simulink model "sedemo_gg1"  (Simulink 7.5)
settings: Solver=ode45  StartTime=0.0  StopTime=10000  RelTol=1e-3
PostLoadFcn:
  | open_system([gcs '/Arrival Process Variance']);
  | open_system([gcs '/Service Process Variance']);
  | open_system([gcs '/Queue Content']);
  | open_system([gcs '/Arrival Rate: Theoretical  vs. Simulation Results']);
undefined symbols (not defined in the file or in its folder): des_attributefunction_support, DiscIntNeverNeededParam
libraries: simulink x6, simeventsattributes2 x3, simeventssink1 x1, simeventsqueue1 x1, simeventstranslate1 x1, simeventsinfo x1, simeventsserver1 x1, simeventsgenerators1 x1
CloseFcn:
  | close_system([gcs '/Arrival Process Variance']);
  | close_system([gcs '/Service Process Variance']);
  | close_system([gcs '/Queue Content']);
  | close_system([gcs '/Arrival Rate: Theoretical  vs. Simulation Results']);
settings Model: Creator=The MathWorks Inc.  ExtModeAutoUpdateStatusClock=off
settings DataIOCC: SaveOutput=off  SignalLogging=off  SaveTime=off
settings OptimizationCC: InitFltsAndDblsToZero=on  BufferReusableBoundary=off
settings DebuggingCC: SignalResolutionControl=TryResolveAllWithWarning  SolverPrmCheckMsg=none  MultiTaskDSMMsg=warning  MultiTaskCondExecSysMsg=none  SigSpecEnsureSampleTimeMsg=none  IntegerOverflowMsg=none  Int32ToFloatConvMsg=none  ParameterDowncastMsg=none  ParameterOverflowMsg=none  ParameterPrecisionLossMsg=none  BusObjectLabelMismatch=none  StrictBusMsg=None
settings RTWCC: IncludeERTFirstTime=on
settings SimEventsCC: propIdentEventSeed=12345678  propDiagAttribOutput=1  propDiagFcnCallOutput=1  propDiagStatOutput=0

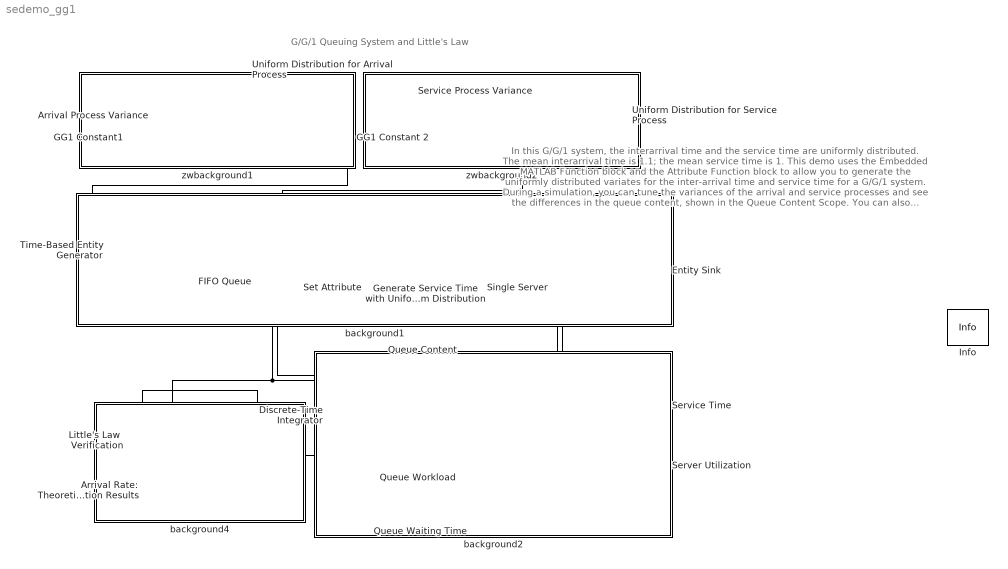
== system sedemo_gg1 ==
  note: G/G/1 Queuing System and Little's Law
  note: In this G/G/1 system, the interarrival time and the
      | service time are uniformly distributed. The mean
      | interarrival time is 1.1; the mean service time is 1.
      |
      | This demo uses the Embedded MATLAB Function
      | block and the Attribute Function block to allow you
      | to generate the  uniformly distributed variates for the
      | inter-arrival time and service time for a G/G/1 system.
      |
      | During a simulation, you can tune the variances of
      | the arrival and service processes and see the
      | differences in the queue content, shown in the Queue
      | Content Scope.
      |
      | You can also verify the Little's law by deriving
      | the arrival rate from average workload and
      | average waiting time. See the Arrival Rate Scope for
      | details.
  Arrival Process Variance : simulink/Math Operations/Slider Gain  SystemSampleTime=-1  low=0  gain=0.3  high=0.40333
  Arrival Rate: Theoretical  vs. Simulation Results : Scope
      settings: YMin=0  YMax=1.1
  Discrete-Time Integrator : DiscreteIntegrator  SampleTime=0.2  OutDataType=sfix(16)  OutScaling=2^0  ICPrevOutput=DiscIntNeverNeededParam  ICPrevScaledInput=DiscIntNeverNeededParam
  Entity Sink : simeventssink1/Entity Sink  Priority=1  SystemSampleTime=-1  AvailableForArrivals=on  StatNumberArrived=Off
  FIFO Queue : simeventsqueue1/FIFO Queue  Priority=1  SystemSampleTime=-1  Capacity=Inf  EnableTOPort=off  StatNumberDeparted=Off  StatNumberInBlock=On  StatPendingEntity=Off  StatAverageWait=On  StatAverageQueueLength=Off  StatNumberTimedout=Off
  "GG1 Constant 2 " : Constant  OutDataType=sfix(16)  OutScaling=2^0
  GG1 Constant1 : Constant  OutDataType=sfix(16)  OutScaling=2^0
  Generate Service Time with Uniform Distribution : Subsystem  LoadFcn=des_attributefunction_support(gcb,'LoadFcn');  StartFcn=des_attributefunction_support(gcb,'StartFcn');  mask(Attribute Function){OutputNamePrefix=out_}
      mask prompts: OutputNamePrefix "Prefix name"
      settings: CopyFcn=des_attributefunction_support(gcb,'CopyFcn');  OpenFcn=des_attributefunction_support(gcb,'OpenFcn');  ErrorFcn=des_error_redirect
      mask Display: image(des_iconLoad('attribFunction.jpg'),'center');
  Info : simeventsinfo/Info  SystemSampleTime=-1
  Little's Law  Verification : Subsystem
      mask Type: Little's Law Evaluation
      mask Description: Evaluate arrival rate from average workload and mean waiting time according to Little's Law. Combine and output this result and the known arrival rate.
      mask Display: disp('Little''s Law\nEvaluation');
  Queue Content : Scope
      settings: YMin=0  YMax=12  SaveName=ScopeData5
  Queue Waiting Time : Display
  Queue Workload : Display
  Server Utilization : Display
  Service Process Variance : simulink/Math Operations/Slider Gain  SystemSampleTime=-1  low=0  gain=0.3  high=0.33333
  Service Time : Display
  Set Attribute : simeventsattributes2/Set Attribute  Priority=1  DialogController=des_ddg_create  DialogControllerArgs=DataTag8  SystemSampleTime=-1  AttributeFrom=Signal port  AttributeName=Variance  AttributeTreatAsVector=1  AttributeValue=1  AttributeCreate=on  StatNumberDeparted=Off  EvaluatedAttributeValue={[]}
  Single Server : simeventsserver1/Single Server  Priority=1  SystemSampleTime=-1  ServiceTimeFrom=Attribute  ServiceTime=1  AttributeName=ServiceTime  PriorityServiceCompletion=1  PermitPreemption=off  SortingAttributeName=PriorityAttributeName  SortingDirection=Ascending  WriteToAttribute=off  ResidualAttributeName=ResidualServiceTime  CreateAttribute=on  EnableTOPort=off  StatNumberDeparted=Off  StatNumberInBlock=Off  StatNumberPreempted=Off  StatPendingEntity=Off  StatAverageWait=On  StatUtilization=On  StatNumberTimedout=Off
  Time-Based Entity Generator : simeventsgenerators1/Entity Generators/Time-Based Entity Generator  Priority=1  DialogController=des_ddg_create  DialogControllerArgs=DataTag11  SystemSampleTime=-1  GenerateEntitiesUpon=Intergeneration time from port t  Distribution=Constant  Minimum=0  Maximum=1  Mean=1  InitialSeed=12345  Period=1  PriorityEntityGeneration=1  GenerateEntityAtSimulationStart=on  ResponseWhenBlocked=Pause generation  ResponseWhenUnblocked=Immediate restart  EntityType=Standard  StatNumberDeparted=Off  StatPendingEntity=Off  StatAverageIntergenerationTime=Off
  Uniform Distribution for Arrival Process : Subsystem  mask(Uniform Distribution for Interarrival Time){seed=85274}
      mask prompts: seed "Initial seed"
      mask help: Output interarrival times according to a uniform distribution. The mean is set to 1.1 and the variance is determined by the input. Output is repeatable for a given seed.
      mask Display: disp('Uniform\nDistribution for\nInterarrival Time');
  Uniform Distribution for Service Process : Subsystem
      mask Display: disp(['Variance ' char(10) 'Validation']);
  background1 : Subsystem
      mask Display: disp('')
  background2 : Subsystem
      mask Display: disp('')
  background4 : Subsystem
      mask Display: disp('')
  zwbackground1 : Subsystem
      mask Display: disp('')
  zwbackground2 : Subsystem
      mask Display: disp('')
  wires:
  FIFO Queue/1 -> Queue Content/1, Discrete-Time Integrator/1
  FIFO Queue/2 -> Queue Waiting Time/1, Little's Law  Verification/2(Waiting Time)
  Arrival Process Variance/1 -> Uniform Distribution for Arrival Process/1(Variance)
  GG1 Constant1/1 -> Arrival Process Variance/1
  Uniform Distribution for Arrival Process/1(Out1) -> Time-Based Entity Generator/1
  Service Process Variance/1 -> Set Attribute/1, Uniform Distribution for Service Process/1(Variance)
  "GG1 Constant 2 "/1 -> Service Process Variance/1
  Discrete-Time Integrator/1 -> Little's Law  Verification/1(Number of  Customers Served), Queue Workload/1
  Single Server/1 -> Service Time/1
  Little's Law  Verification/1(Out1) -> Arrival Rate: Theoretical  vs. Simulation Results/1
  Single Server/2 -> Server Utilization/1
  connections:
  Time-Based Entity Generator/RConn1 -- FIFO Queue/LConn1
  Single Server/RConn1 -- Entity Sink/LConn1
  Set Attribute/LConn1 -- FIFO Queue/RConn1
  Generate Service Time with Uniform Distribution/LConn1 -- Set Attribute/RConn1
  Single Server/LConn1 -- Generate Service Time with Uniform Distribution/RConn1

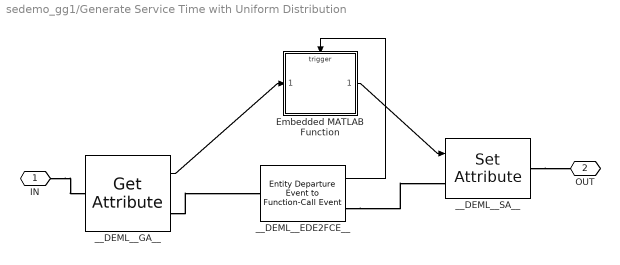
== system sedemo_gg1/Generate Service Time with Uniform Distribution ==
  Embedded MATLAB Function : Stateflow chart  TreatAsAtomicUnit=on
      settings: PropExecContextOutsideSubsystem=on
  __DEML__EDE2FCE__ : simeventstranslate1/Entity Departure Event to Function-Call Event  Priority=1  SystemSampleTime=-1  TimingFunctionCallF1=Before entity departure  EnableE1Port=off  EnableF2Port=off  TimingFunctionCallF2=Before entity departure  EnableE2Port=off  StatNumberDeparted=Off  StatNumberF1Calls=Off  StatNumberF2Calls=Off  IsInsideAFB=on
  __DEML__GA__ : simeventsattributes2/Get Attribute  Priority=1  DialogController=des_ddg_create  DialogControllerArgs=DataTag4  SystemSampleTime=-1  AttributeName=Variance  AttributeMissing=Error  AttributeDefaultValue=1  AttributeSendTiming=Before entity departure  AttributeTreatAsVector=1  StatNumberDeparted=Off  EvaluatedDefaultAttributeValue={[]}
  __DEML__SA__ : simeventsattributes2/Set Attribute  Priority=1  DialogController=des_ddg_create  DialogControllerArgs=DataTag6  SystemSampleTime=-1  AttributeFrom=Signal port  AttributeName=ServiceTime  AttributeTreatAsVector=1  AttributeValue=1  AttributeCreate=on  StatNumberDeparted=Off  EvaluatedAttributeValue={[]}
  IN : PMIOPort  Port=1  Side=Left
  OUT : PMIOPort  Port=2  Side=Right
  wires:
  __DEML__EDE2FCE__/1 -> Embedded MATLAB Function/Trigger
  __DEML__GA__/1 -> Embedded MATLAB Function/1(Variance)
  Embedded MATLAB Function/1(out_ServiceTime) -> __DEML__SA__/1
  connections:
  __DEML__EDE2FCE__/RConn1 -- __DEML__SA__/LConn1
  __DEML__GA__/RConn1 -- __DEML__EDE2FCE__/LConn1
  IN/RConn1 -- __DEML__GA__/LConn1
  __DEML__SA__/RConn1 -- OUT/RConn1

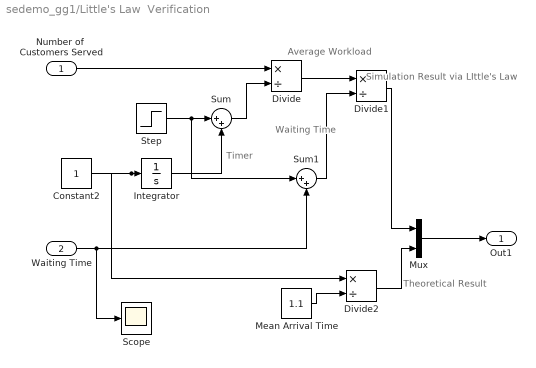
== system sedemo_gg1/Little's Law  Verification ==
  note: Simulation Result
      | via LIttle's Law
  note: Theoretical Result
  note: Timer
  note: Average
      | Workload
  note: Waiting
      | Time
  Number of  Customers Served : Inport  OutDataType=sfix(16)  OutScaling=2^0
  Waiting Time : Inport  Port=2  OutDataType=sfix(16)  OutScaling=2^0
  Constant2 : Constant  OutDataType=sfix(16)  OutScaling=2^0
  Divide : Product  Inputs=*/  OutDataType=sfix(16)  OutScaling=2^-10
  Divide1 : Product  Inputs=*/  OutDataType=sfix(16)  OutScaling=2^-10
  Divide2 : Product  Inputs=*/  OutDataType=sfix(16)  OutScaling=2^-10
  Integrator : Integrator
  Mean Arrival Time : Constant  Value=1.1  OutDataType=sfix(16)  OutScaling=2^0
  Mux : Mux  Inputs=2
  Scope : Scope
  Step : Step  Time=50  Before=1  After=0  SampleTime=0
  Sum : Sum  Inputs=|++  OutDataType=sfix(16)  OutScaling=2^0
  Sum1 : Sum  Inputs=|++  OutDataType=sfix(16)  OutScaling=2^0
  Out1 : Outport  OutDataType=sfix(16)  OutScaling=2^0
  wires:
  Constant2/1 -> Divide2/1, Integrator/1
  Divide/1 -> Divide1/1
  Mean Arrival Time/1 -> Divide2/2
  Divide2/1 -> Mux/2
  Mux/1 -> Out1/1
  Divide1/1 -> Mux/1
  Step/1 -> Sum/1, Sum1/1
  Integrator/1 -> Sum/2
  Sum/1 -> Divide/2
  Waiting Time/1 -> Sum1/2, Scope/1
  Sum1/1 -> Divide1/2
  Number of  Customers Served/1 -> Divide/1

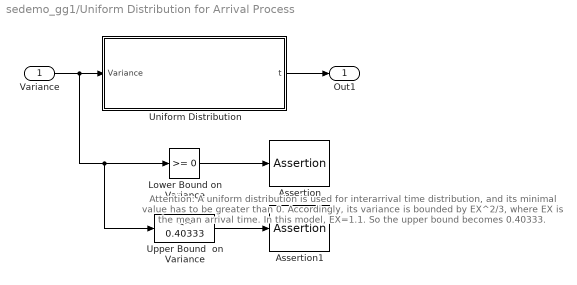
== system sedemo_gg1/Uniform Distribution for Arrival Process ==
  note: Attention: A uniform distribution is used
      | for interarrival time distribution, and its
      | minimal value has to be greater than 0.
      | Accordingly, its variance is bounded by
      | EX^2/3, where EX is the mean arrival
      | time. In this model, EX=1.1. So the
      | upper bound becomes 0.40333.
  Variance : Inport  OutDataType=sfix(16)  OutScaling=2^0
  Assertion : Assertion  Enabled=on
  Assertion1 : Assertion  Enabled=on
  Lower Bound on Variance : simulink/Logic and Bit Operations/Compare To Constant  SystemSampleTime=-1  relop=>=  const=0  LogicOutDataTypeMode=uint8  ZeroCross=off
  Uniform Distribution : Stateflow chart  TreatAsAtomicUnit=on
  "Upper Bound  on Variance " : simulink/Logic and Bit Operations/Compare To Constant  SystemSampleTime=-1  relop=<=  const=0.40333  LogicOutDataTypeMode=uint8  ZeroCross=off
  Out1 : Outport  OutDataType=sfix(16)  OutScaling=2^0
  wires:
  Uniform Distribution/1(t) -> Out1/1
  "Upper Bound  on Variance "/1 -> Assertion1/1
  Lower Bound on Variance/1 -> Assertion/1
  Variance/1 -> Uniform Distribution/1(Variance), "Upper Bound  on Variance "/1, Lower Bound on Variance/1

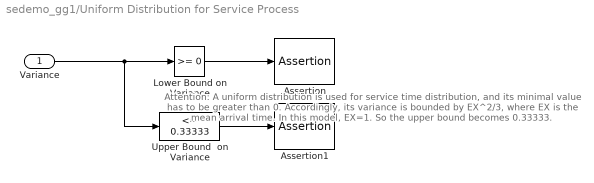
== system sedemo_gg1/Uniform Distribution for Service Process ==
  note: Attention: A uniform distribution is used
      | for service time distribution, and its
      | minimal value has to be greater than 0.
      | Accordingly, its variance is bounded by
      | EX^2/3, where EX is the mean arrival
      | time. In this model, EX=1. So the
      | upper bound becomes 0.33333.
  Variance : Inport  OutDataType=sfix(16)  OutScaling=2^0
  Assertion : Assertion  Enabled=on
  Assertion1 : Assertion  Enabled=on
  Lower Bound on Variance : simulink/Logic and Bit Operations/Compare To Constant  SystemSampleTime=-1  relop=>=  const=0  LogicOutDataTypeMode=uint8  ZeroCross=off
  "Upper Bound  on Variance " : simulink/Logic and Bit Operations/Compare To Constant  SystemSampleTime=-1  relop=<=  const=0.33333  LogicOutDataTypeMode=uint8  ZeroCross=off
  wires:
  Variance/1 -> Lower Bound on Variance/1, "Upper Bound  on Variance "/1
  Lower Bound on Variance/1 -> Assertion/1
  "Upper Bound  on Variance "/1 -> Assertion1/1

== system sedemo_gg1/background1 ==

== system sedemo_gg1/background2 ==

== system sedemo_gg1/background4 ==

== system sedemo_gg1/zwbackground1 ==
  note: This subsystem is empty

== system sedemo_gg1/zwbackground2 ==
  note: This subsystem is empty

== matlab function Generate Service Time with Uniform Distribution/Embedded MATLAB Function ==
  data: Variance input double; out_ServiceTime output double
  events: trigger input FUNCTION_CALL_EVENT
function out_ServiceTime  = GenServiceTime(Variance)
% This function generates uniformly distributed service time.

persistent initialize_seed;
% Initialize the seed for the 
% first call
if(isempty(initialize_seed))
    rand('seed',96286);
    initialize_seed = 1;
end

MeanServiceTime = 1;

% The lower limit for the uniform distribution is 0;
% b is the upper limit of the uniform distribution 
% for the given variance
b = 2*sqrt(3*Variance);

% Center the distribution around zero: b(rng-1/2)
% Shift the distribution obtain samples with 
% the mean arrival time
out_ServiceTime = b*(rand-1/2) + MeanServiceTime;

== matlab function Uniform Distribution for Arrival Process/Uniform Distribution ==
  data: t output double; Variance input double; seed parameter double
function t = GenInterArrivalTime(Variance, seed)
% This function generates uniformly distributed interarrival time
% distributed in [0,b] interval with the specified variance and 
% mean arrival time

persistent initialize_seed;
% Initialize the seed for the 
% first call
if(isempty(initialize_seed))
    rand('seed',seed);
    initialize_seed = 1;
end

MeanArrivalTime = 1.1;
% The lower limit for the uniform distribution is 0;
% b is the upper limit of the uniform distribution
% for the given variance
b = 2*sqrt(3*Variance);

% Center the distribution around zero: b(rng-1/2)
% Shift the distribution to get the mean arrival time
t = b*(rand-1/2) + MeanArrivalTime;
